simulink subsystem "Model_airdrag"  (R2023a)
settings: Solver=VariableStepAuto  StartTime=0.0  StopTime=10.0  RelTol=1e-3
undefined symbols (not defined in the file): C_D_drone, S_x, S_y, S_z
settings Model: Creator=raduserseniuc  LastModifiedBy=raduserseniuc

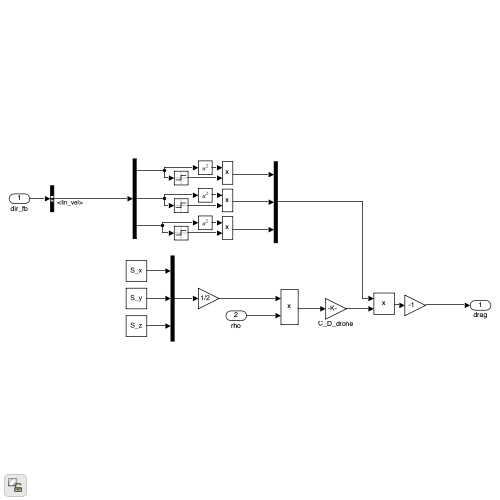
[thumbnail: Simulink's stored preview of the top-level diagram]
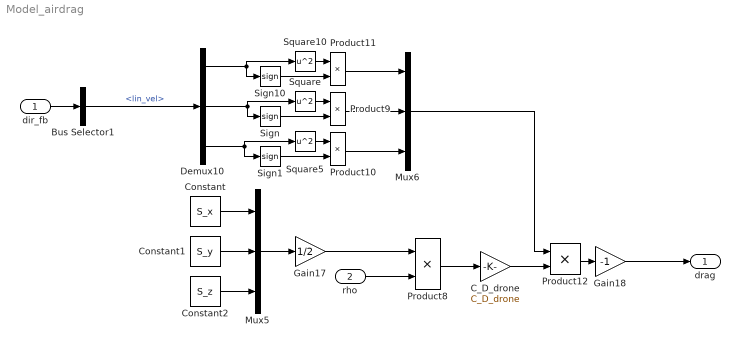
== system Model_airdrag ==
  dir_fb : Inport
  rho : Inport  Port=2
  Bus Selector1 : BusSelector  OutputSignals=lin_vel
  C_D_drone : Gain  Gain=C_D_drone
  Constant : Constant  Value=S_x
  Constant1 : Constant  Value=S_y
  Constant2 : Constant  Value=S_z
  Demux10 : Demux  Outputs=3
  Gain17 : Gain  Gain=1/2
  Gain18 : Gain  Gain=-1
  Mux5 : Mux  Inputs=3
  Mux6 : Mux  Inputs=3
  Product{8..12} (5 alike) : Product
  Sign : Signum
  Sign1 : Signum
  Sign10 : Signum
  Square : Math  Operator=square
  Square10 : Math  Operator=square
  Square5 : Math  Operator=square
  drag : Outport
  wires:
  Mux6/1 -> Product12/1
  Demux10/2 -> Square/1, Sign/1
  Gain17/1 -> Product8/1
  Product12/1 -> Gain18/1
  Product11/1 -> Mux6/1
  Demux10/3 -> Square5/1, Sign1/1
  Square/1 -> Product9/1
  rho/1 -> Product8/2
  Bus Selector1/1 -> Demux10/1  "<lin_vel>"
  Demux10/1 -> Square10/1, Sign10/1
  Sign1/1 -> Product10/2
  Constant2/1 -> Mux5/3
  Sign/1 -> Product9/2
  Square5/1 -> Product10/1
  Product8/1 -> C_D_drone/1
  Product10/1 -> Mux6/3
  Product9/1 -> Mux6/2
  Mux5/1 -> Gain17/1
  Sign10/1 -> Product11/2
  C_D_drone/1 -> Product12/2
  Constant/1 -> Mux5/1
  Constant1/1 -> Mux5/2
  Gain18/1 -> drag/1
  Square10/1 -> Product11/1
  dir_fb/1 -> Bus Selector1/1
